simulink model "adarbha_HW7_sim"  (Simulink 7.7)
settings: Solver=ode45  StartTime=0.0  StopTime=1000  RelTol=1e-3
InitFcn:
  | Init_File_IC_Engine_HW_7_adarbha
values from neighbouring files (symbols this model uses):
  Area = 2.4    [Init_File_IC_Engine_HW_7_JEB.m]
  Cd = 0.44    [Init_File_IC_Engine_HW_7_JEB.m]
  density_gasoline = 726    [Init_File_IC_Engine_HW_7_JEB.m]
  fr = 0.01    [Init_File_IC_Engine_HW_7_JEB.m]
  FUEL_FLOW = [0.2022	0.2508	0.2922	0.6462	0.6588	0.6786	0.8658	0.909	0.9738	1.107	1.0854	0.963	1.1214	1.4184	1.1772	1.2276	1.2546	1.2924	1.494	1.5264	1.422	2.475	3.0402	2.9214	2.322	1.4886	0.5832	0.0018	0.0036	0.0054 ... (first row only)    [Init_File_IC_Engine_HW_7_JEB.m]
  K = 44.67    [Init_File_IC_Engine_HW_7_JEB.m]
  kph_to_m_sec = 1000/3600    (= 0.277777777778)    [Init_File_IC_Engine_HW_7_JEB.m]
  Mass = Weight/g    (= 1904.17940877)    [Init_File_IC_Engine_HW_7_JEB.m]
  Nd = 3.73    [Init_File_IC_Engine_HW_7_JEB.m]
  Nt1 = 2.2    [Init_File_IC_Engine_HW_7_JEB.m]
  Nt2 = 1.64    [Init_File_IC_Engine_HW_7_JEB.m]
  Nt3 = 1.28    [Init_File_IC_Engine_HW_7_JEB.m]
  Nt4 = 1.0    (= 1)    [Init_File_IC_Engine_HW_7_JEB.m]
  OMEGA_ICE = [1000.000	1146.552	1293.103	1439.655	1586.207	1732.759	1879.310	2025.862	2172.414	2318.966	2465.517	2612.069	2758.621	2905.172	3051.724	3198.276	3344.828	3491.379	3637.931	3784.483	3931.034	4077.586	4224.138	4370.690	4517.241	4663.793	4810.345	4956.897	5103.448	5250.000]    [Init_File_IC_Engine_HW_7_JEB.m]
  R_Wheel = 0.318    [Init_File_IC_Engine_HW_7_JEB.m]
  rho = 1.224    [Init_File_IC_Engine_HW_7_JEB.m]
  Time = xlsread('Malibu_20100929_highway_Baseline.xls','A:A')    [Init_File_IC_Engine_HW_7_JEB.m]
  TORQUE_ICE = [0.000	10.552	21.103	31.655	42.206	52.758	63.310	73.861	84.415	94.966	105.518	116.069	126.621	137.173	147.724	158.276	168.827	179.379	189.931	200.482	211.034	221.585	232.139	242.690	253.242	263.794	274.345	284.897	295.448	306.000]    [Init_File_IC_Engine_HW_7_JEB.m]
  Velocity_kph = xlsread('Malibu_20100929_highway_Baseline.xls','B:B')    [Init_File_IC_Engine_HW_7_JEB.m]
  Weight = 18680    [Init_File_IC_Engine_HW_7_JEB.m]
settings Model: Creator=jebeard  LastModifiedBy=Arjun

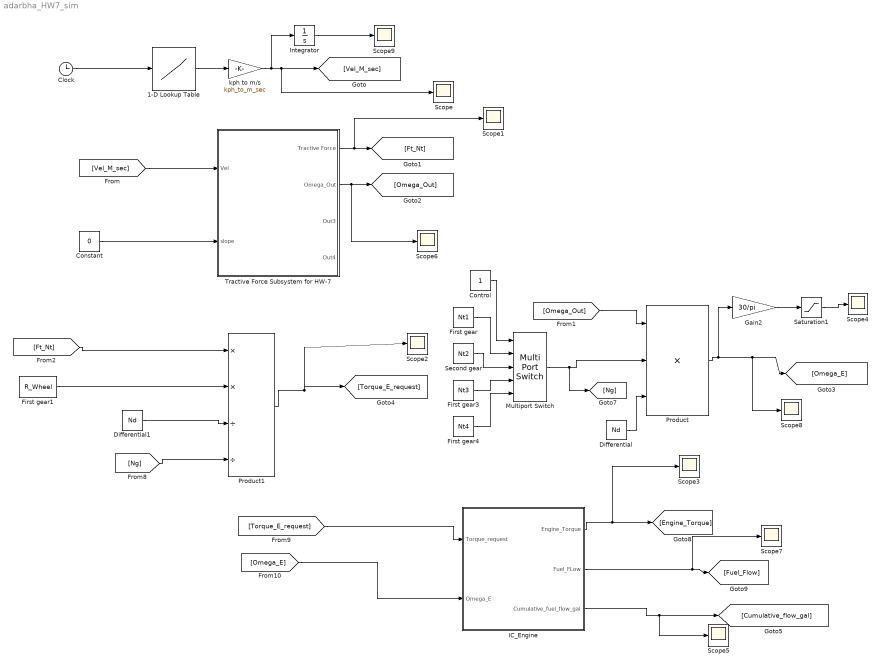
== system adarbha_HW7_sim ==
  1-D Lookup Table : Lookup_n-D  NumberOfTableDimensions=1  BreakpointsForDimension1=Time  Table=Velocity_kph  RndMeth=Simplest  InputSameDT=on
  Clock : Clock
      settings: Decimation=10
  Constant : Constant  Value=0
  Control : Constant
  Differential : Constant  Value=Nd
  Differential1 : Constant  Value=Nd
  First gear : Constant  Value=Nt1
  First gear1 : Constant  Value=R_Wheel
  First gear3 : Constant  Value=Nt3
  First gear4 : Constant  Value=Nt4
  Gain2 : Gain  Gain=30/pi
  IC_Engine : Subsystem
  Integrator : Integrator
  Multiport Switch : MultiPortSwitch  Inputs=4  zeroidx=off
  Product : Product  Inputs=3  RndMeth=Zero
  Product1 : Product  Inputs=**//  RndMeth=Zero
  Saturation1 : Saturate  UpperLimit=Inf  LowerLimit=1000
  Scope{,1..9} (10 alike) : Scope
      Scope2 settings: SaveName=ScopeData2
      Scope3 settings: SaveName=ScopeData3
      Scope4 settings: SaveName=ScopeData6
      Scope5 settings: SaveName=ScopeData8
      Scope6 settings: SaveName=ScopeData11
      Scope7 settings: SaveName=ScopeData12
      Scope8 settings: SaveName=ScopeData13
      Scope9 settings: SaveName=ScopeData15
  Second gear : Constant  Value=Nt2
  Tractive Force Subsystem for HW-7 : Subsystem  TreatAsAtomicUnit=on
  kph to m/s : Gain  Gain=kph_to_m_sec
  wires:
  Clock/1 -> 1-D Lookup Table/1
  1-D Lookup Table/1 -> kph to m/s/1
  kph to m/s/1 -> [Vel_M_sec], Scope/1, Integrator/1
  [Vel_M_sec] -> Tractive Force Subsystem for HW-7/1(Vel)
  Constant/1 -> Tractive Force Subsystem for HW-7/2(slope)
  Tractive Force Subsystem for HW-7/1(Tractive Force) -> [Ft_Nt], Scope1/1
  Tractive Force Subsystem for HW-7/2(Omega_Out) -> [Omega_Out], Scope6/1
  [Omega_Out] -> Product/1
  Differential/1 -> Product/3
  Product/1 -> Gain2/1, [Omega_E], Scope8/1
  [Ft_Nt] -> Product1/1
  Differential1/1 -> Product1/3
  First gear1/1 -> Product1/2
  Product1/1 -> [Torque_E_request], Scope2/1
  [Ng] -> Product1/4
  First gear/1 -> Multiport Switch/2
  Second gear/1 -> Multiport Switch/3
  First gear3/1 -> Multiport Switch/4
  First gear4/1 -> Multiport Switch/5
  Control/1 -> Multiport Switch/1
  Multiport Switch/1 -> Product/2, [Ng]
  Gain2/1 -> Saturation1/1
  Saturation1/1 -> Scope4/1
  IC_Engine/1(Engine_Torque) -> [Engine_Torque], Scope3/1
  [Torque_E_request] -> IC_Engine/1(Torque_request)
  [Omega_E] -> IC_Engine/2(Omega_E)
  IC_Engine/2(Fuel_FLow) -> [Fuel_Flow], Scope7/1
  IC_Engine/3(Cumulative_fuel_flow_gal) -> [Cumulative_flow_gal], Scope5/1
  Integrator/1 -> Scope9/1

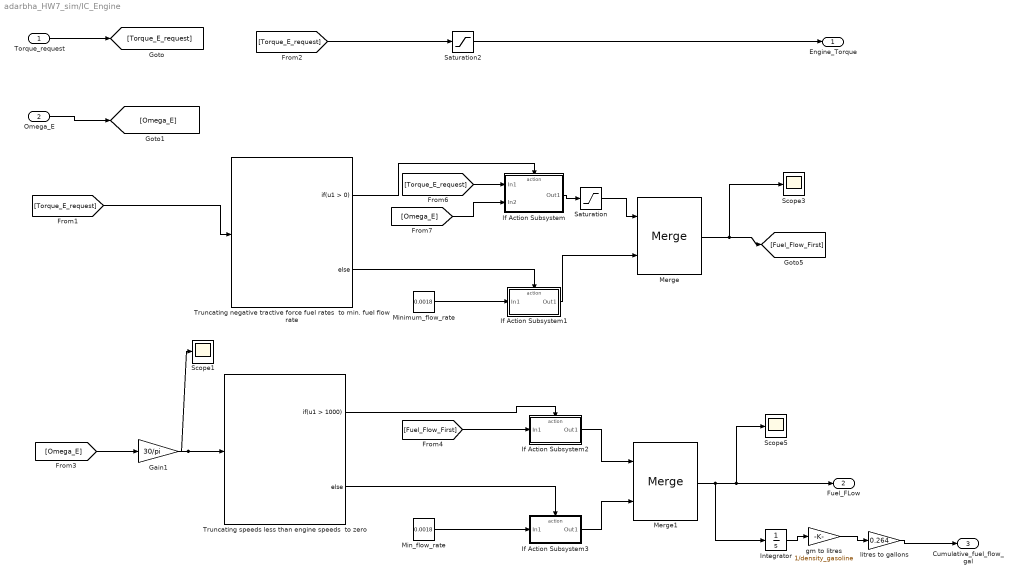
== system adarbha_HW7_sim/IC_Engine ==
  Torque_request : Inport
  Omega_E : Inport  Port=2
  Gain1 : Gain  Gain=30/pi
  If Action Subsystem : Subsystem  TreatAsAtomicUnit=on
  If Action Subsystem1 : Subsystem  TreatAsAtomicUnit=on
  If Action Subsystem2 : Subsystem  TreatAsAtomicUnit=on
  If Action Subsystem3 : Subsystem  TreatAsAtomicUnit=on
  Integrator : Integrator
  Merge : Merge
  Merge1 : Merge
  Min_flow_rate : Constant  Value=0.0018
  Minimum_flow_rate : Constant  Value=0.0018
  Saturation : Saturate  UpperLimit=Inf  LowerLimit=0.0018
  Saturation2 : Saturate  UpperLimit=Inf  LowerLimit=0
  Scope1 : Scope
      settings: SaveName=ScopeData14
  Scope3 : Scope
      settings: SaveName=ScopeData9
  Scope5 : Scope
      settings: SaveName=ScopeData10
  Truncating negative tractive force fuel rates  to min. fuel flow rate : If
  Truncating speeds less than engine speeds  to zero : If  IfExpression=u1 > 1000
  gm to litres : Gain  Gain=1/density_gasoline
  litres to gallons : Gain  Gain=0.264
  Engine_Torque : Outport
  Fuel_FLow : Outport  Port=2
  Cumulative_fuel_flow_gal : Outport  Port=3
  wires:
  Saturation2/1 -> Engine_Torque/1
  Minimum_flow_rate/1 -> If Action Subsystem1/1(In1)
  Merge/1 -> [Fuel_Flow_First], Scope3/1
  [Torque_E_request] -> Truncating negative tractive force fuel rates  to min. fuel flow rate/1
  [Torque_E_request] -> If Action Subsystem/1(In1)
  [Omega_E] -> If Action Subsystem/2(In2)
  Truncating negative tractive force fuel rates  to min. fuel flow rate/1 -> If Action Subsystem/Action
  Truncating negative tractive force fuel rates  to min. fuel flow rate/2 -> If Action Subsystem1/Action
  If Action Subsystem1/1(Out1) -> Merge/2
  If Action Subsystem/1(Out1) -> Saturation/1
  Saturation/1 -> Merge/1
  [Omega_E] -> Gain1/1
  Truncating speeds less than engine speeds  to zero/1 -> If Action Subsystem2/Action
  [Fuel_Flow_First] -> If Action Subsystem2/1(In1)
  Min_flow_rate/1 -> If Action Subsystem3/1(In1)
  Truncating speeds less than engine speeds  to zero/2 -> If Action Subsystem3/Action
  If Action Subsystem2/1(Out1) -> Merge1/1
  If Action Subsystem3/1(Out1) -> Merge1/2
  Merge1/1 -> Scope5/1, Fuel_FLow/1, Integrator/1
  Gain1/1 -> Truncating speeds less than engine speeds  to zero/1, Scope1/1
  Torque_request/1 -> [Torque_E_request]
  Omega_E/1 -> [Omega_E]
  [Torque_E_request] -> Saturation2/1
  Integrator/1 -> gm to litres/1
  gm to litres/1 -> litres to gallons/1
  litres to gallons/1 -> Cumulative_fuel_flow_gal/1

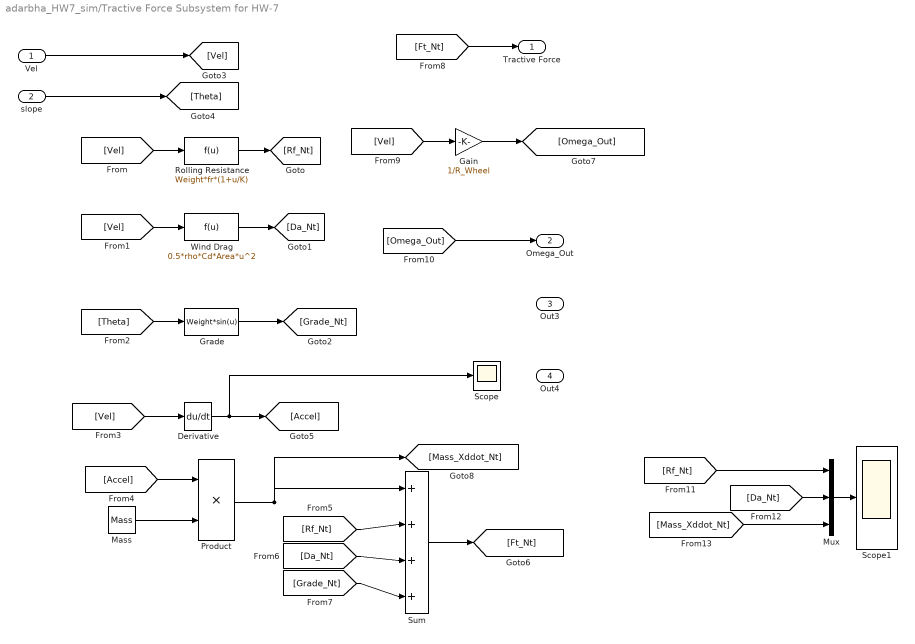
== system adarbha_HW7_sim/Tractive Force Subsystem for HW-7 ==
  Vel : Inport
  slope : Inport  Port=2
  Derivative : Derivative
  Gain : Gain  Gain=1/R_Wheel
  Grade : Fcn  Expr=Weight*sin(u)
  Mass : Constant  Value=Mass
  Mux : Mux  Inputs=3
  Product : Product  RndMeth=Zero
  Rolling Resistance : Fcn  Expr=Weight*fr*(1+u/K)
  Scope : Scope
      settings: SaveName=ScopeData4
  Scope1 : Scope
      settings: SaveName=ScopeData5
  Sum : Sum  Inputs=|+|+|+|+|
  Wind Drag : Fcn  Expr=0.5*rho*Cd*Area*u^2
  Tractive Force : Outport
  Omega_Out : Outport  Port=2
  Out3 : Outport  Port=3
  Out4 : Outport  Port=4
  wires:
  [Vel] -> Rolling Resistance/1
  Rolling Resistance/1 -> [Rf_Nt]
  [Vel] -> Wind Drag/1
  Wind Drag/1 -> [Da_Nt]
  [Theta] -> Grade/1
  Grade/1 -> [Grade_Nt]
  Vel/1 -> [Vel]
  slope/1 -> [Theta]
  [Vel] -> Derivative/1
  Derivative/1 -> [Accel], Scope/1
  Mass/1 -> Product/2
  [Accel] -> Product/1
  Product/1 -> Sum/1, [Mass_Xddot_Nt]
  [Rf_Nt] -> Sum/2
  [Da_Nt] -> Sum/3
  [Grade_Nt] -> Sum/4
  Sum/1 -> [Ft_Nt]
  [Ft_Nt] -> Tractive Force/1
  [Vel] -> Gain/1
  Gain/1 -> [Omega_Out]
  [Omega_Out] -> Omega_Out/1
  [Da_Nt] -> Mux/2
  [Rf_Nt] -> Mux/1
  Mux/1 -> Scope1/1
  [Mass_Xddot_Nt] -> Mux/3

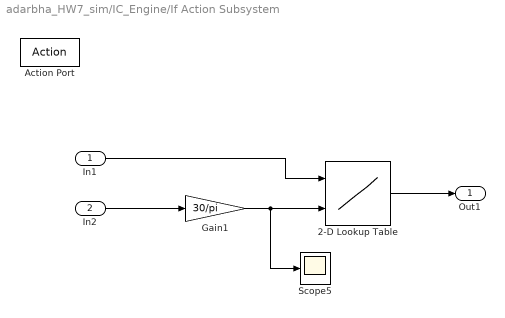
== system adarbha_HW7_sim/IC_Engine/If Action Subsystem ==
  In1 : Inport
  In2 : Inport  Port=2
  Action Port : ActionPort  ActionType=then
  2-D Lookup Table : Lookup_n-D  BreakpointsForDimension1=TORQUE_ICE  BreakpointsForDimension2=OMEGA_ICE  Table=FUEL_FLOW  RndMeth=Simplest  InputSameDT=on
  Gain1 : Gain  Gain=30/pi
  Scope5 : Scope
      settings: SaveName=ScopeData7
  Out1 : Outport
  wires:
  Gain1/1 -> 2-D Lookup Table/2, Scope5/1
  In2/1 -> Gain1/1
  In1/1 -> 2-D Lookup Table/1
  2-D Lookup Table/1 -> Out1/1

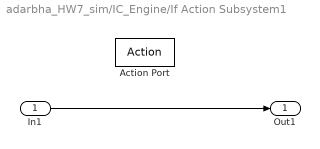
== system adarbha_HW7_sim/IC_Engine/If Action Subsystem1 ==
  In1 : Inport
  Action Port : ActionPort  ActionType=else
  Out1 : Outport
  wires:
  In1/1 -> Out1/1

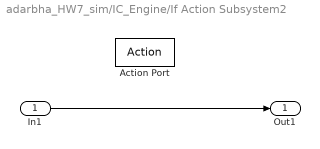
== system adarbha_HW7_sim/IC_Engine/If Action Subsystem2 ==
  In1 : Inport
  Action Port : ActionPort  ActionType=then
  Out1 : Outport
  wires:
  In1/1 -> Out1/1

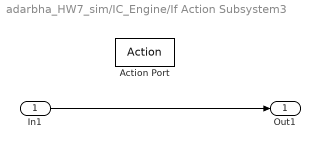
== system adarbha_HW7_sim/IC_Engine/If Action Subsystem3 ==
  In1 : Inport
  Action Port : ActionPort  ActionType=else
  Out1 : Outport
  wires:
  In1/1 -> Out1/1
